simulink model "testGrinding"  (R2023a)
settings: Solver=VariableStepAuto  StartTime=0.0  StopTime=10.0  RelTol=1e-3
libraries: NSA_DEVS_SINKS_ATOMIC x6, NSA_DEVS_SOURCES_ATOMIC x2, NSA_DEVS_LOGISTICS_ATOMIC x1, ProductionLineLib_CM x1
settings Model: Creator=peter  LastModifiedBy=david

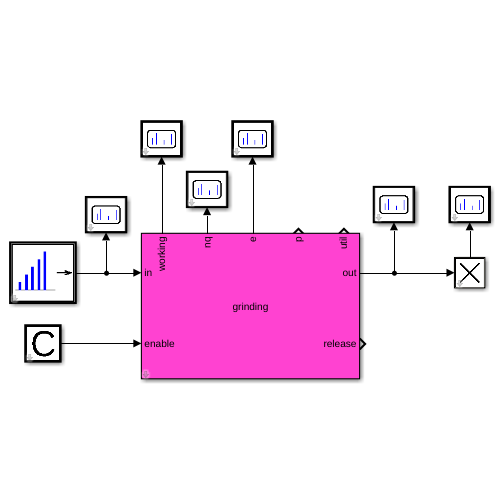
[thumbnail: Simulink's stored preview of the top-level diagram]
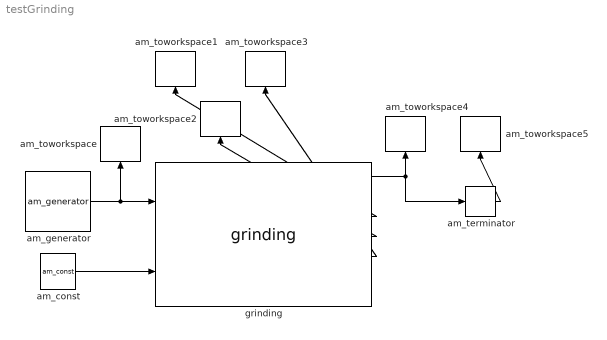
== system testGrinding ==
  am_const : NSA_DEVS_SOURCES_ATOMIC/am_const  value="\"1\""  sendTime=[0,1]  tau=[0,1]  debug=0
      settings: SourceProductName=NSA_DEVS
  am_generator : NSA_DEVS_SOURCES_ATOMIC/am_generator  tG=300  n0=1  nG=30  tau=[0,1]  debug=0
      settings: SourceProductName=NSA_DEVS
  am_terminator : NSA_DEVS_LOGISTICS_ATOMIC/am_terminator  tau=[0,1]  debug=0
      settings: SourceProductName=NSA_DEVS
  am_toworkspace : NSA_DEVS_SINKS_ATOMIC/am_toworkspace  varname="\"o1\""  t0=0  format="\"vector\""  tau=[0,5]  debug=0
      settings: SourceProductName=NSA_DEVS
  am_toworkspace1 : NSA_DEVS_SINKS_ATOMIC/am_toworkspace  varname="\"o2\""  t0=0  format="\"vector\""  tau=[0,5]  debug=0
      settings: SourceProductName=NSA_DEVS
  am_toworkspace2 : NSA_DEVS_SINKS_ATOMIC/am_toworkspace  varname="\"o3\""  t0=0  format="\"vector\""  tau=[0,5]  debug=0
      settings: SourceProductName=NSA_DEVS
  am_toworkspace3 : NSA_DEVS_SINKS_ATOMIC/am_toworkspace  varname="\"o4\""  t0=0  format="\"vector\""  tau=[0,5]  debug=0
      settings: SourceProductName=NSA_DEVS
  am_toworkspace4 : NSA_DEVS_SINKS_ATOMIC/am_toworkspace  varname="\"o5\""  t0=0  format="\"vector\""  tau=[0,5]  debug=0
      settings: SourceProductName=NSA_DEVS
  am_toworkspace5 : NSA_DEVS_SINKS_ATOMIC/am_toworkspace  varname="\"o6\""  t0=0  format="\"vector\""  tau=[0,5]  debug=0
      settings: SourceProductName=NSA_DEVS
  grinding : ProductionLineLib_CM/grinding  vfr1=0.48  vfr2=0.19  vfr3=0.03  vc=30  max_fifo=400  tauInt=[0,100]  tauCont=[0,100]  tau=[0,1]  debug=0
  wires:
  am_terminator/1 -> am_toworkspace5/1
  am_generator/1 -> am_toworkspace/1, grinding/1
  am_const/1 -> grinding/2
  grinding/1 -> am_terminator/1, am_toworkspace4/1
  grinding/3 -> am_toworkspace1/1
  grinding/4 -> am_toworkspace2/1
  grinding/5 -> am_toworkspace3/1
